simulink model "gm_lab3_step9"  (R2019b)
settings: Solver=VariableStepAuto  StartTime=0.0  StopTime=stop_time  RelTol=1e-3
InitFcn:
  | sm_callback_init
StopFcn:
  | sm_callback_stop
undefined symbols (not defined in the file or in its folder): mp
libraries: hdlsllib x10, simulink x3
(part 2 of 2)

== system gm_lab3_step9/dataplane/Avalon Data Processing/Left Channel Processing/Signal Energy Monitor/LED_Driver/LED_persistence_control3/Chart/Chart ==
  LED_trigger : Inport  OutDataTypeStr=boolean  PortDimensions=1  SampleTime=1.01725260416667e-08
  count_reached : Inport  Port=2  OutDataTypeStr=boolean  PortDimensions=1  SampleTime=1.01725260416667e-08
  Chart : Stateflow chart  BlockKeywords=__PRM__SERIALIZED__DATA__:Stateflow Chart,Stateflow Diagram  TreatAsAtomicUnit=on
  LED_signal : Outport  InitialOutput=0
  counter_reset : Outport  Port=2  InitialOutput=0
  wires:
  Chart/2(counter_reset) -> counter_reset/1
  Chart/1(LED_signal) -> LED_signal/1
  count_reached/1 -> Chart/2(count_reached)
  LED_trigger/1 -> Chart/1(LED_trigger)

== system gm_lab3_step9/dataplane/Avalon Data Processing/Left Channel Processing/Signal Energy Monitor/LED_Driver/LED_persistence_control4/Chart/Chart ==
  LED_trigger : Inport  OutDataTypeStr=boolean  PortDimensions=1  SampleTime=1.01725260416667e-08
  count_reached : Inport  Port=2  OutDataTypeStr=boolean  PortDimensions=1  SampleTime=1.01725260416667e-08
  Chart : Stateflow chart  BlockKeywords=__PRM__SERIALIZED__DATA__:Stateflow Chart,Stateflow Diagram  TreatAsAtomicUnit=on
  LED_signal : Outport  InitialOutput=0
  counter_reset : Outport  Port=2  InitialOutput=0
  wires:
  Chart/2(counter_reset) -> counter_reset/1
  Chart/1(LED_signal) -> LED_signal/1
  count_reached/1 -> Chart/2(count_reached)
  LED_trigger/1 -> Chart/1(LED_trigger)

== system gm_lab3_step9/dataplane/Avalon Data Processing/Left Channel Processing/Signal Energy Monitor/LED_Driver/LED_persistence_control5/Chart/Chart ==
  LED_trigger : Inport  OutDataTypeStr=boolean  PortDimensions=1  SampleTime=1.01725260416667e-08
  count_reached : Inport  Port=2  OutDataTypeStr=boolean  PortDimensions=1  SampleTime=1.01725260416667e-08
  Chart : Stateflow chart  BlockKeywords=__PRM__SERIALIZED__DATA__:Stateflow Chart,Stateflow Diagram  TreatAsAtomicUnit=on
  LED_signal : Outport  InitialOutput=0
  counter_reset : Outport  Port=2  InitialOutput=0
  wires:
  Chart/2(counter_reset) -> counter_reset/1
  Chart/1(LED_signal) -> LED_signal/1
  count_reached/1 -> Chart/2(count_reached)
  LED_trigger/1 -> Chart/1(LED_trigger)

== system gm_lab3_step9/dataplane/Avalon Data Processing/Left Channel Processing/Signal Energy Monitor/LED_Driver/LED_persistence_control6/Chart/Chart ==
  LED_trigger : Inport  OutDataTypeStr=boolean  PortDimensions=1  SampleTime=1.01725260416667e-08
  count_reached : Inport  Port=2  OutDataTypeStr=boolean  PortDimensions=1  SampleTime=1.01725260416667e-08
  Chart : Stateflow chart  BlockKeywords=__PRM__SERIALIZED__DATA__:Stateflow Chart,Stateflow Diagram  TreatAsAtomicUnit=on
  LED_signal : Outport  InitialOutput=0
  counter_reset : Outport  Port=2  InitialOutput=0
  wires:
  Chart/2(counter_reset) -> counter_reset/1
  Chart/1(LED_signal) -> LED_signal/1
  count_reached/1 -> Chart/2(count_reached)
  LED_trigger/1 -> Chart/1(LED_trigger)

== system gm_lab3_step9/dataplane/Avalon Data Processing/Left Channel Processing/Signal Energy Monitor/LED_Driver/LED_persistence_control7/Chart/Chart ==
  LED_trigger : Inport  OutDataTypeStr=boolean  PortDimensions=1  SampleTime=1.01725260416667e-08
  count_reached : Inport  Port=2  OutDataTypeStr=boolean  PortDimensions=1  SampleTime=1.01725260416667e-08
  Chart : Stateflow chart  BlockKeywords=__PRM__SERIALIZED__DATA__:Stateflow Chart,Stateflow Diagram  TreatAsAtomicUnit=on
  LED_signal : Outport  InitialOutput=0
  counter_reset : Outport  Port=2  InitialOutput=0
  wires:
  Chart/2(counter_reset) -> counter_reset/1
  Chart/1(LED_signal) -> LED_signal/1
  count_reached/1 -> Chart/2(count_reached)
  LED_trigger/1 -> Chart/1(LED_trigger)

== stateflow chart gm_lab3_step9/dataplane/Avalon Data Processing/Left Channel Processing/Signal Energy Monitor/LED_Driver/LED_persistence_control1/Chart/Chart/Chart ==
  settings: executeAtInitialization=1
  state LED_off
    entry: LED_signal=false;
    entry: counter_reset=true;
  state LED_on
    entry: LED_signal=true;
    entry: counter_reset=false;
  (default) -> LED_off
  LED_off -> LED_on : [LED_trigger==1]
  LED_on -> LED_off : [count_reached==1]
  data: LED_trigger input; count_reached input; LED_signal output; counter_reset output

== stateflow chart gm_lab3_step9/dataplane/Avalon Data Processing/Left Channel Processing/Signal Energy Monitor/LED_Driver/LED_persistence_control/Chart/Chart/Chart ==
  settings: executeAtInitialization=1
  state LED_off
    entry: LED_signal=false;
    entry: counter_reset=true;
  state LED_on
    entry: LED_signal=true;
    entry: counter_reset=false;
  (default) -> LED_off
  LED_off -> LED_on : [LED_trigger==1]
  LED_on -> LED_off : [count_reached==1]
  data: LED_trigger input; count_reached input; LED_signal output; counter_reset output

== stateflow chart gm_lab3_step9/dataplane/Avalon Data Processing/Left Channel Processing/Signal Energy Monitor/LED_Driver/LED_persistence_control2/Chart/Chart/Chart ==
  settings: executeAtInitialization=1
  state LED_off
    entry: LED_signal=false;
    entry: counter_reset=true;
  state LED_on
    entry: LED_signal=true;
    entry: counter_reset=false;
  (default) -> LED_off
  LED_off -> LED_on : [LED_trigger==1]
  LED_on -> LED_off : [count_reached==1]
  data: LED_trigger input; count_reached input; LED_signal output; counter_reset output

== stateflow chart gm_lab3_step9/dataplane/Avalon Data Processing/Left Channel Processing/Signal Energy Monitor/LED_Driver/LED_persistence_control3/Chart/Chart/Chart ==
  settings: executeAtInitialization=1
  state LED_off
    entry: LED_signal=false;
    entry: counter_reset=true;
  state LED_on
    entry: LED_signal=true;
    entry: counter_reset=false;
  (default) -> LED_off
  LED_off -> LED_on : [LED_trigger==1]
  LED_on -> LED_off : [count_reached==1]
  data: LED_trigger input; count_reached input; LED_signal output; counter_reset output

== stateflow chart gm_lab3_step9/dataplane/Avalon Data Processing/Left Channel Processing/Signal Energy Monitor/LED_Driver/LED_persistence_control4/Chart/Chart/Chart ==
  settings: executeAtInitialization=1
  state LED_off
    entry: LED_signal=false;
    entry: counter_reset=true;
  state LED_on
    entry: LED_signal=true;
    entry: counter_reset=false;
  (default) -> LED_off
  LED_off -> LED_on : [LED_trigger==1]
  LED_on -> LED_off : [count_reached==1]
  data: LED_trigger input; count_reached input; LED_signal output; counter_reset output

== stateflow chart gm_lab3_step9/dataplane/Avalon Data Processing/Left Channel Processing/Signal Energy Monitor/LED_Driver/LED_persistence_control5/Chart/Chart/Chart ==
  settings: executeAtInitialization=1
  state LED_off
    entry: LED_signal=false;
    entry: counter_reset=true;
  state LED_on
    entry: LED_signal=true;
    entry: counter_reset=false;
  (default) -> LED_off
  LED_off -> LED_on : [LED_trigger==1]
  LED_on -> LED_off : [count_reached==1]
  data: LED_trigger input; count_reached input; LED_signal output; counter_reset output

== stateflow chart gm_lab3_step9/dataplane/Avalon Data Processing/Left Channel Processing/Signal Energy Monitor/LED_Driver/LED_persistence_control6/Chart/Chart/Chart ==
  settings: executeAtInitialization=1
  state LED_off
    entry: LED_signal=false;
    entry: counter_reset=true;
  state LED_on
    entry: LED_signal=true;
    entry: counter_reset=false;
  (default) -> LED_off
  LED_off -> LED_on : [LED_trigger==1]
  LED_on -> LED_off : [count_reached==1]
  data: LED_trigger input; count_reached input; LED_signal output; counter_reset output

== stateflow chart gm_lab3_step9/dataplane/Avalon Data Processing/Left Channel Processing/Signal Energy Monitor/LED_Driver/LED_persistence_control7/Chart/Chart/Chart ==
  settings: executeAtInitialization=1
  state LED_off
    entry: LED_signal=false;
    entry: counter_reset=true;
  state LED_on
    entry: LED_signal=true;
    entry: counter_reset=false;
  (default) -> LED_off
  LED_off -> LED_on : [LED_trigger==1]
  LED_on -> LED_off : [count_reached==1]
  data: LED_trigger input; count_reached input; LED_signal output; counter_reset output
